simulink model "RUN_2nd_ASE_370C_MiniProject1_simulink"  (R2018b)
settings: Solver=VariableStepAuto  StartTime=0.0  StopTime=15  RelTol=1e-3
InitFcn:
  | RUN_1st_ASE_370C_MiniProject1
values from neighbouring files (symbols this model uses):
  A = [0 1 0 0 ... (first row only)    [ASE_370C_HW5_Controls.m]    (also in RUN_1st_ASE_370C_MiniProject1.m = [0 0 1 0)
  Apert = A + .02*randn(4,4)    [RUN_1st_ASE_370C_MiniProject1.m]
  B = [0; 0; 1/m; r/J]    [RUN_1st_ASE_370C_MiniProject1.m]
  C = [1 0 0 0]    [ASE_370C_HW5_Controls.m]    (also in ASE_370C_HW6_Controls.m = [1 0]; RUN_1st_ASE_370C_MiniProject1.m)
  K = [-110 2 113 1]    [ASE_370C_HW5_Controls.m]    (also in ASE_370C_MinProj2_main.m = 20; RUN_1st_ASE_370C_MiniProject1.m = place(A,B,eigs))
  k_i = 10')    [ASE_370C_MiniProj3_test.m]    (also in RUN_1st_ASE_370C_MiniProject1.m = K_int(end))
  k_r = double(vpasolve(G_ry == -C_ry / A_ry * B_ry_sym, krsym))    [RUN_1st_ASE_370C_MiniProject1.m]
  KK = K_int(1:4)    [RUN_1st_ASE_370C_MiniProject1.m]
  x0 = 0    [ASE_370C_HW3_Controls.m]    (also in RUN_1st_ASE_370C_MiniProject1.m = zeros(4,1))
CloseFcn:
  | ASE_370C_MiniProject1_Plots
settings Model: Creator=kenda  LastModifiedBy=kenda

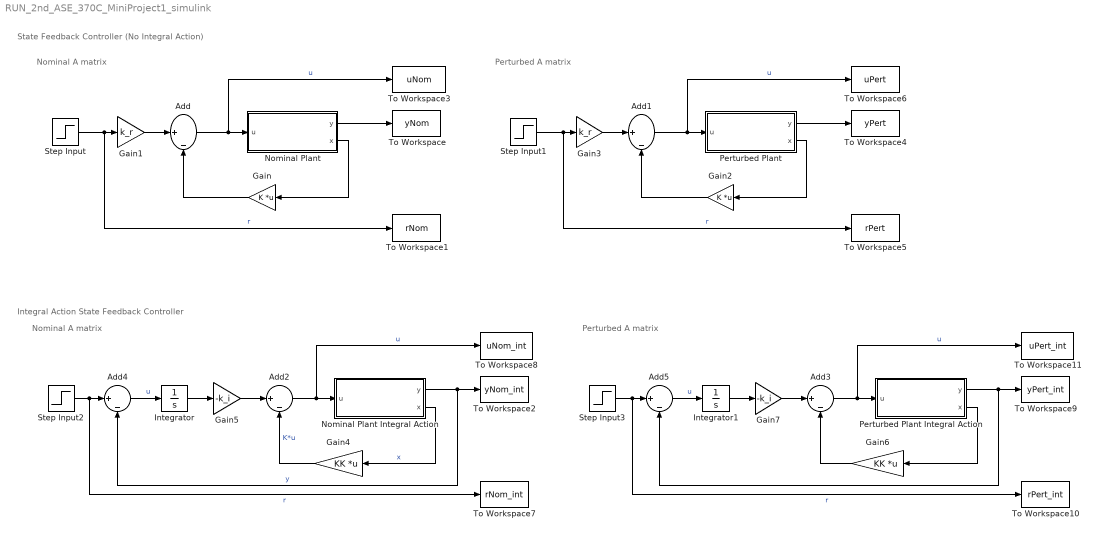
== system RUN_2nd_ASE_370C_MiniProject1_simulink ==
  note: State Feedback Controller (No Integral Action)
  note: Nominal A matrix
  note: Perturbed A matrix
  note: Integral Action State Feedback Controller
  note: Nominal A matrix
  note: Perturbed A matrix
  Add{,1..5} (6 alike) : Sum  Inputs=||+|-
  Gain : Gain  Gain=K  Multiplication=Matrix(K*u)
  Gain1 : Gain  Gain=k_r
  Gain2 : Gain  Gain=K  Multiplication=Matrix(K*u)
  Gain3 : Gain  Gain=k_r
  Gain4 : Gain  Gain=KK  Multiplication=Matrix(K*u)
  Gain5 : Gain  Gain=-k_i
  Gain6 : Gain  Gain=KK  Multiplication=Matrix(K*u)
  Gain7 : Gain  Gain=-k_i
  Integrator : Integrator
  Integrator1 : Integrator
  Nominal Plant : Subsystem
  Nominal Plant Integral Action : Subsystem
  Perturbed Plant : Subsystem
  Perturbed Plant Integral Action : Subsystem
  Step Input{,1..3} (4 alike) : Step  SampleTime=0
  To Workspace : ToWorkspace  VariableName=yNom  SaveFormat=Timeseries  SampleTime=-1
  To Workspace1 : ToWorkspace  VariableName=rNom  SaveFormat=Timeseries  SampleTime=-1
  To Workspace10 : ToWorkspace  VariableName=rPert_int  SaveFormat=Timeseries  SampleTime=-1
  To Workspace11 : ToWorkspace  VariableName=uPert_int  SaveFormat=Timeseries  SampleTime=-1
  To Workspace2 : ToWorkspace  VariableName=yNom_int  SaveFormat=Timeseries  SampleTime=-1
  To Workspace3 : ToWorkspace  VariableName=uNom  SaveFormat=Timeseries  SampleTime=-1
  To Workspace4 : ToWorkspace  VariableName=yPert  SaveFormat=Timeseries  SampleTime=-1
  To Workspace5 : ToWorkspace  VariableName=rPert  SaveFormat=Timeseries  SampleTime=-1
  To Workspace6 : ToWorkspace  VariableName=uPert  SaveFormat=Timeseries  SampleTime=-1
  To Workspace7 : ToWorkspace  VariableName=rNom_int  SaveFormat=Timeseries  SampleTime=-1
  To Workspace8 : ToWorkspace  VariableName=uNom_int  SaveFormat=Timeseries  SampleTime=-1
  To Workspace9 : ToWorkspace  VariableName=yPert_int  SaveFormat=Timeseries  SampleTime=-1
  wires:
  Step Input/1 -> To Workspace1/1, Gain1/1  "r"
  Gain1/1 -> Add/1
  Add/1 -> To Workspace3/1, Nominal Plant/1(u)  "u"
  Nominal Plant/2(x) -> Gain/1
  Gain/1 -> Add/2
  Nominal Plant/1(y) -> To Workspace/1
  Perturbed Plant/1(y) -> To Workspace4/1
  Perturbed Plant/2(x) -> Gain2/1
  Gain3/1 -> Add1/1
  Step Input1/1 -> To Workspace5/1, Gain3/1  "r"
  Gain2/1 -> Add1/2
  Add1/1 -> To Workspace6/1, Perturbed Plant/1(u)  "u"
  Nominal Plant Integral Action/1(y) -> To Workspace2/1, Add4/2  "y"
  Gain4/1 -> Add2/2  "K*u"
  Nominal Plant Integral Action/2(x) -> Gain4/1  "x"
  Gain5/1 -> Add2/1
  Add2/1 -> To Workspace8/1, Nominal Plant Integral Action/1(u)  "u"
  Integrator/1 -> Gain5/1
  Step Input2/1 -> To Workspace7/1, Add4/1  "r"
  Add4/1 -> Integrator/1  "u"
  Perturbed Plant Integral Action/2(x) -> Gain6/1
  Perturbed Plant Integral Action/1(y) -> To Workspace9/1, Add5/2
  Gain7/1 -> Add3/1
  Gain6/1 -> Add3/2
  Step Input3/1 -> To Workspace10/1, Add5/1  "r"
  Add5/1 -> Integrator1/1  "u"
  Integrator1/1 -> Gain7/1
  Add3/1 -> To Workspace11/1, Perturbed Plant Integral Action/1(u)  "u"

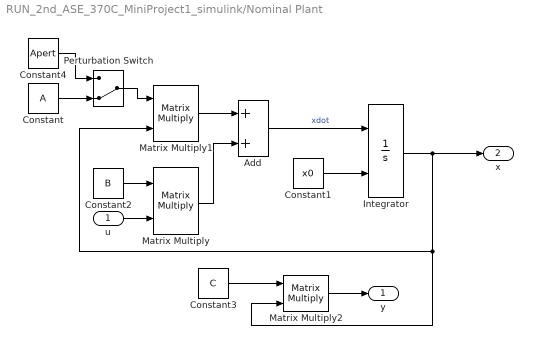
== system RUN_2nd_ASE_370C_MiniProject1_simulink/Nominal Plant ==
  u : Inport
  Add : Sum
  Constant : Constant  Value=A  VectorParams1D=off
  Constant1 : Constant  Value=x0  VectorParams1D=off
  Constant2 : Constant  Value=B  VectorParams1D=off
  Constant3 : Constant  Value=C  VectorParams1D=off
  Constant4 : Constant  Value=Apert
  Integrator : Integrator  InitialConditionSource=external
  Matrix Multiply : Product  Multiplication=Matrix(*)
  Matrix Multiply1 : Product  Multiplication=Matrix(*)
  Matrix Multiply2 : Product  Multiplication=Matrix(*)
  Perturbation Switch : ManualSwitch  CurrentSetting=0
  y : Outport
  x : Outport  Port=2
  wires:
  Constant/1 -> Perturbation Switch/2
  Integrator/1 -> Matrix Multiply2/2, Matrix Multiply1/2, x/1
  Constant1/1 -> Integrator/2
  Add/1 -> Integrator/1  "xdot"
  Constant2/1 -> Matrix Multiply/1
  u/1 -> Matrix Multiply/2
  Matrix Multiply/1 -> Add/2
  Matrix Multiply1/1 -> Add/1
  Constant3/1 -> Matrix Multiply2/1
  Matrix Multiply2/1 -> y/1
  Constant4/1 -> Perturbation Switch/1
  Perturbation Switch/1 -> Matrix Multiply1/1

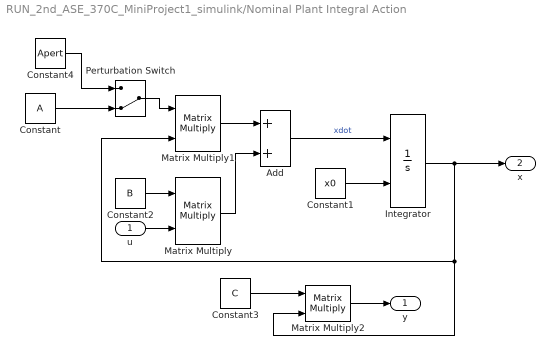
== system RUN_2nd_ASE_370C_MiniProject1_simulink/Nominal Plant Integral Action ==
  u : Inport
  Add : Sum
  Constant : Constant  Value=A  VectorParams1D=off
  Constant1 : Constant  Value=x0  VectorParams1D=off
  Constant2 : Constant  Value=B  VectorParams1D=off
  Constant3 : Constant  Value=C  VectorParams1D=off
  Constant4 : Constant  Value=Apert
  Integrator : Integrator  InitialConditionSource=external
  Matrix Multiply : Product  Multiplication=Matrix(*)
  Matrix Multiply1 : Product  Multiplication=Matrix(*)
  Matrix Multiply2 : Product  Multiplication=Matrix(*)
  Perturbation Switch : ManualSwitch  CurrentSetting=0
  y : Outport
  x : Outport  Port=2
  wires:
  Constant/1 -> Perturbation Switch/2
  Integrator/1 -> Matrix Multiply2/2, Matrix Multiply1/2, x/1
  Constant1/1 -> Integrator/2
  Add/1 -> Integrator/1  "xdot"
  Constant2/1 -> Matrix Multiply/1
  u/1 -> Matrix Multiply/2
  Matrix Multiply/1 -> Add/2
  Matrix Multiply1/1 -> Add/1
  Constant3/1 -> Matrix Multiply2/1
  Matrix Multiply2/1 -> y/1
  Constant4/1 -> Perturbation Switch/1
  Perturbation Switch/1 -> Matrix Multiply1/1

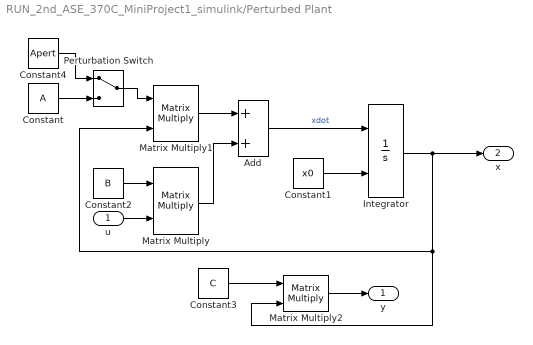
== system RUN_2nd_ASE_370C_MiniProject1_simulink/Perturbed Plant ==
  u : Inport
  Add : Sum
  Constant : Constant  Value=A  VectorParams1D=off
  Constant1 : Constant  Value=x0  VectorParams1D=off
  Constant2 : Constant  Value=B  VectorParams1D=off
  Constant3 : Constant  Value=C  VectorParams1D=off
  Constant4 : Constant  Value=Apert
  Integrator : Integrator  InitialConditionSource=external
  Matrix Multiply : Product  Multiplication=Matrix(*)
  Matrix Multiply1 : Product  Multiplication=Matrix(*)
  Matrix Multiply2 : Product  Multiplication=Matrix(*)
  Perturbation Switch : ManualSwitch
  y : Outport
  x : Outport  Port=2
  wires:
  Constant/1 -> Perturbation Switch/2
  Integrator/1 -> Matrix Multiply2/2, Matrix Multiply1/2, x/1
  Constant1/1 -> Integrator/2
  Add/1 -> Integrator/1  "xdot"
  Constant2/1 -> Matrix Multiply/1
  u/1 -> Matrix Multiply/2
  Matrix Multiply/1 -> Add/2
  Matrix Multiply1/1 -> Add/1
  Constant3/1 -> Matrix Multiply2/1
  Matrix Multiply2/1 -> y/1
  Constant4/1 -> Perturbation Switch/1
  Perturbation Switch/1 -> Matrix Multiply1/1

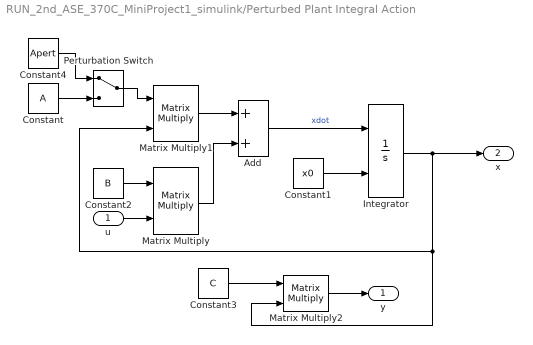
== system RUN_2nd_ASE_370C_MiniProject1_simulink/Perturbed Plant Integral Action ==
  u : Inport
  Add : Sum
  Constant : Constant  Value=A  VectorParams1D=off
  Constant1 : Constant  Value=x0  VectorParams1D=off
  Constant2 : Constant  Value=B  VectorParams1D=off
  Constant3 : Constant  Value=C  VectorParams1D=off
  Constant4 : Constant  Value=Apert
  Integrator : Integrator  InitialConditionSource=external
  Matrix Multiply : Product  Multiplication=Matrix(*)
  Matrix Multiply1 : Product  Multiplication=Matrix(*)
  Matrix Multiply2 : Product  Multiplication=Matrix(*)
  Perturbation Switch : ManualSwitch
  y : Outport
  x : Outport  Port=2
  wires:
  Constant/1 -> Perturbation Switch/2
  Integrator/1 -> Matrix Multiply2/2, Matrix Multiply1/2, x/1
  Constant1/1 -> Integrator/2
  Add/1 -> Integrator/1  "xdot"
  Constant2/1 -> Matrix Multiply/1
  u/1 -> Matrix Multiply/2
  Matrix Multiply/1 -> Add/2
  Matrix Multiply1/1 -> Add/1
  Constant3/1 -> Matrix Multiply2/1
  Matrix Multiply2/1 -> y/1
  Constant4/1 -> Perturbation Switch/1
  Perturbation Switch/1 -> Matrix Multiply1/1
